simulink model "acc_decision_core"  (R2024b)
settings: Solver=FixedStepDiscrete  StartTime=0.0  StopTime=inf  FixedStep=0.05  RelTol=1e-3
InitFcn:
  | load('decision_lookup_data.mat');
model workspace (MAT data in the model file):
  command_bp = [0 1 2 3 4 5 6 7]
  control_enabled_table = [1  1  1  1  1  1  0  0; 0  1  1  0  0  0  0  0; 0  1  0  0  0  0  0  0; 0  0  0  0  0  0  0  0]
  decision_raw_table = [-1  1  2  3  4  7  8  8; 8  5  6  8  8  8  8  8; 8  5  8  8  8  8  8  8; 8  8  8  8  8  8  8  8]
  decision_table = [-1  1  2  3  4  7  8  8; 8  5  6  8  8  8  8  8; 8  5  8  8  8  8  8  8; 8  8  8  8  8  8  8  8]
  next_state_table = [0  0  0  0  0  0  1  1; 1  0  0  1  1  1  1  1; 2  0  2  2  2  2  2  2; 3  3  3  3  3  3  3  3]
  side_effect_table = [0  0  0  0  0  0  0  0; 0  0  0  0  0  0  0  0; 0  1  0  0  0  0  0  0; 0  0  0  0  0  0  0  0]
  state_bp = [0 1 2 3]
undefined symbols (not defined in the file or in its folder): f
libraries: instrumentlib x2
settings Model: Creator=aiden  LastModifiedBy=aiden

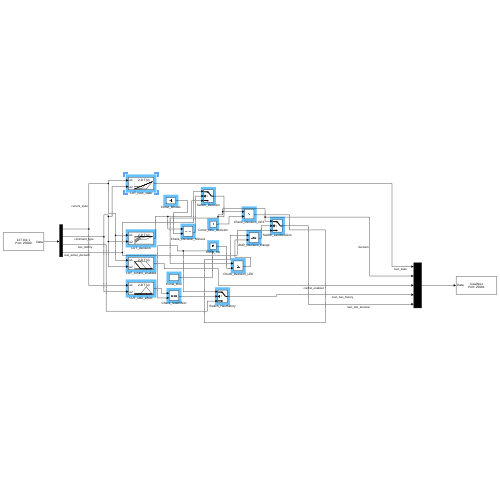
[thumbnail: Simulink's stored preview of the top-level diagram]
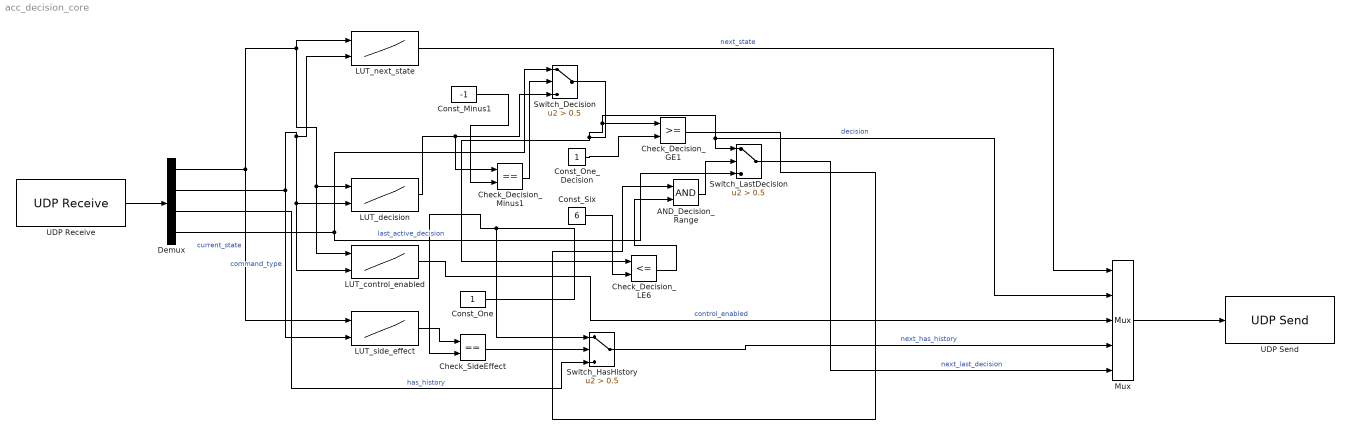
== system acc_decision_core ==
  AND_Decision_Range : Logic  AllPortsSameDT=off  OutDataTypeStr=boolean
  Check_Decision_GE1 : RelationalOperator  OutDataTypeStr=boolean  RndMeth=Simplest  InputSameDT=off
  Check_Decision_LE6 : RelationalOperator  Operator=<=  OutDataTypeStr=boolean  RndMeth=Simplest  InputSameDT=off
  Check_Decision_Minus1 : RelationalOperator  Operator===  OutDataTypeStr=boolean  RndMeth=Simplest  InputSameDT=off
  Check_SideEffect : RelationalOperator  Operator===  OutDataTypeStr=boolean  RndMeth=Simplest  InputSameDT=off
  Const_Minus1 : Constant  Value=-1
  Const_One : Constant
  Const_One_Decision : Constant
  Const_Six : Constant  Value=6
  Demux : Demux
  LUT_control_enabled : Lookup_n-D  BreakpointsForDimension1=state_bp  BreakpointsForDimension2=command_bp  BreakpointsForDimension3=[5, 7]  Table=control_enabled_table  InternalRulePriority=Speed  RndMeth=Simplest
      settings: InputPortMap=u0,u1
  LUT_decision : Lookup_n-D  BreakpointsForDimension1=state_bp  BreakpointsForDimension2=command_bp  BreakpointsForDimension3=[5, 7]  Table=decision_table  InternalRulePriority=Speed  RndMeth=Simplest
      settings: InputPortMap=u0,u1
  LUT_next_state : Lookup_n-D  BreakpointsForDimension1=state_bp  BreakpointsForDimension2=command_bp  BreakpointsForDimension3=[5, 7]  Table=next_state_table  InternalRulePriority=Speed  RndMeth=Simplest
      settings: InputPortMap=u0,u1
  LUT_side_effect : Lookup_n-D  BreakpointsForDimension1=state_bp  BreakpointsForDimension2=command_bp  BreakpointsForDimension3=[5, 7]  Table=side_effect_table  InternalRulePriority=Speed  RndMeth=Simplest
      settings: InputPortMap=u0,u1
  Mux : Mux  Inputs=5
  Switch_Decision : Switch  Criteria=u2 > Threshold  Threshold=0.5  SaturateOnIntegerOverflow=off  InputSameDT=off
  Switch_HasHistory : Switch  Criteria=u2 > Threshold  Threshold=0.5  SaturateOnIntegerOverflow=off  InputSameDT=off
  Switch_LastDecision : Switch  Criteria=u2 > Threshold  Threshold=0.5  SaturateOnIntegerOverflow=off  InputSameDT=off
  UDP Receive : instrumentlib/UDP Receive  LocalAddress=127.0.0.1  LocalPort=25000  EnablePortSharing=off  Host=localhost  Port=9090  GetLatestData=on  DataSize=[ 4, 1 ]  DataType=double  ASCIIFormatting=%f,  Terminator=LF  CustomTerminator=10  ByteOrder=little-endian  EnableBlockingMode=on  Timeout=20  SampleTime=-1  SimulateUsing=Interpreted execution
  UDP Send : instrumentlib/UDP Send  Host=localhost  Port=25001  LocalAddress=127.0.0.1  LocalPort=25001  EnablePortSharing=on  OutputDatagramPacketSize=512  ByteOrder=little-endian  EnableBlockingMode=off  SimulateUsing=Interpreted execution
  wires:
  LUT_decision/1 -> Check_Decision_Minus1/1, Switch_Decision/3
  Const_Minus1/1 -> Check_Decision_Minus1/2
  Check_Decision_Minus1/1 -> Switch_Decision/2
  LUT_side_effect/1 -> Check_SideEffect/1
  Const_One/1 -> Check_SideEffect/2, Switch_HasHistory/1
  Check_SideEffect/1 -> Switch_HasHistory/2
  Switch_Decision/1 -> Switch_LastDecision/1, Mux/2, Check_Decision_GE1/1, Check_Decision_LE6/1  "decision"
  Const_One_Decision/1 -> Check_Decision_GE1/2
  Const_Six/1 -> Check_Decision_LE6/2
  Check_Decision_GE1/1 -> AND_Decision_Range/1
  Check_Decision_LE6/1 -> AND_Decision_Range/2
  AND_Decision_Range/1 -> Switch_LastDecision/2
  LUT_next_state/1 -> Mux/1  "next_state"
  LUT_control_enabled/1 -> Mux/3  "control_enabled"
  Switch_LastDecision/1 -> Mux/5  "next_last_decision"
  UDP Receive/1 -> Demux/1
  Demux/1 -> LUT_decision/1, LUT_control_enabled/1, LUT_next_state/1, LUT_side_effect/1  "current_state"
  Demux/2 -> LUT_decision/2, LUT_control_enabled/2, LUT_next_state/2, LUT_side_effect/2  "command_type"
  Demux/3 -> Switch_HasHistory/3  "has_history"
  Demux/4 -> Switch_LastDecision/3, Switch_Decision/1  "last_active_decision"
  Switch_HasHistory/1 -> Mux/4  "next_has_history"
  Mux/1 -> UDP Send/1
